simulink model "plant_fuzzy"  (R2020a)
settings: Solver=VariableStepAuto  StartTime=0.0  StopTime=200  RelTol=1e-3
values from neighbouring files (symbols this model uses):
  Ca = 0.005    [reproduce_examples.m]
  Cb = 0.005    [reproduce_examples.m]
  dt = 0.05    [reproduce_examples.m]
  fA = 2    [reproduce_examples.m]
  use_step = 1    [reproduce_examples.m]
  V = 3    [reproduce_examples.m]
libraries: simulink x2, fuzblock x1
settings Model: Creator=salvatore  LastModifiedBy=salvatore
settings DataIOCC: SaveFormat=Array  OutputSaveName=pH, valve

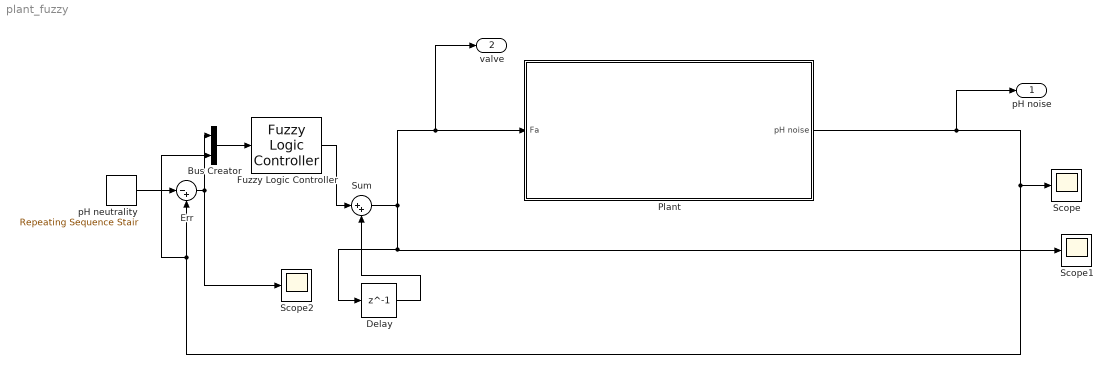
== system plant_fuzzy ==
  Bus Creator : BusCreator  Inputs=2
  Delay : Delay  DelayLength=1  InitialCondition=0
  Err : Sum  Inputs=|-+
  Fuzzy Logic Controller : fuzblock/Fuzzy Logic  Controller  FIS='fuzzy_ph.fis'  OutputSampleNumber=101  DataType=double  FuzzifiedInputs=off  RuleFiringStrengths=off  RuleOutputs=off  AggregatedOutputs=off  SimulateUsing=Interpreted execution  OutOfRangeInputValueMessage=warning  NoRuleFiredMessage=warning  EmptyOutputFuzzySetMessage=warning
  Plant : Subsystem
  Scope : Scope
  Scope1 : Scope
  Scope2 : Scope
  Sum : Sum  Inputs=|++
  pH neutrality : simulink/Sources/Repeating Sequence Stair  OutValues=reference  tsamp=time_ref  OutMin=[]  OutMax=[]  OutDataTypeStr=double  OutputDataTypeScalingMode=double  OutDataType=fixdt(0,8)  ConRadixGroup=Best Precision: Vector-wise  OutScaling=2^-12
  pH noise : Outport  SignalName=ph_noise
  valve : Outport  Port=2  SignalName=valve
  wires:
  pH neutrality/1 -> Err/1
  Sum/1 -> Delay/1, Scope1/1, valve/1, Plant/1(Fa)
  Fuzzy Logic Controller/1 -> Sum/1
  Delay/1 -> Sum/2
  Plant/1(pH noise) -> pH noise/1, Bus Creator/2, Err/2, Scope/1
  Err/1 -> Bus Creator/1, Scope2/1
  Bus Creator/1 -> Fuzzy Logic Controller/1

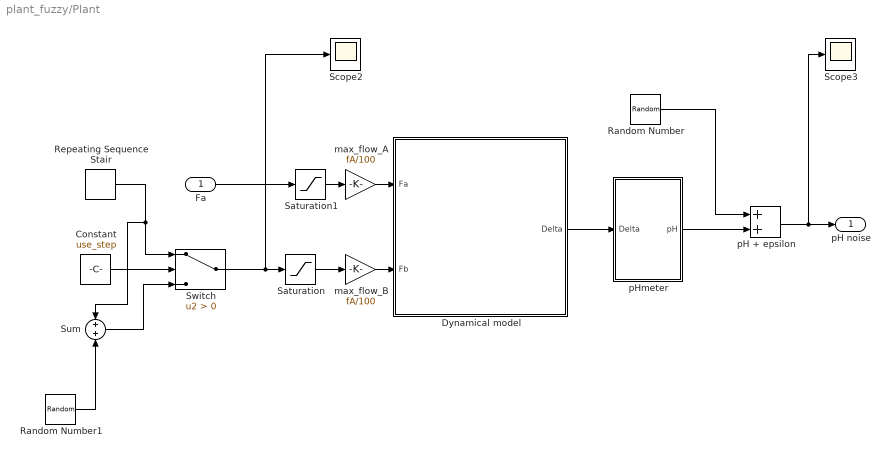
== system plant_fuzzy/Plant ==
  Fa : Inport
  Constant : Constant  Value=use_step
  Dynamical model : Subsystem
  Random Number : RandomNumber  Variance=0.01  SampleTime=dt
  Random Number1 : RandomNumber  Variance=4  SampleTime=1
  Repeating Sequence Stair : simulink/Sources/Repeating Sequence Stair  OutValues=out_valv  tsamp=time_valv  OutMin=[]  OutMax=[]  OutDataTypeStr=double  OutputDataTypeScalingMode=double  OutDataType=fixdt(0,8)  ConRadixGroup=Best Precision: Vector-wise  OutScaling=2^-12
  Saturation : Saturate  UpperLimit=100  LowerLimit=0
  Saturation1 : Saturate  UpperLimit=100  LowerLimit=0
  Scope2 : Scope
  Scope3 : Scope
  Sum : Sum  Inputs=+|+
  Switch : Switch  Criteria=u2 > Threshold
  max_flow_A : Gain  Gain=fA/100
  max_flow_B : Gain  Gain=fA/100
  pH + epsilon : Sum
  pHmeter : Subsystem
  pH noise : Outport
  wires:
  max_flow_A/1 -> Dynamical model/1(Fa)
  max_flow_B/1 -> Dynamical model/2(Fb)
  pH + epsilon/1 -> Scope3/1, pH noise/1
  pHmeter/1(pH) -> pH + epsilon/2
  Saturation1/1 -> max_flow_A/1
  Random Number/1 -> pH + epsilon/1
  Saturation/1 -> max_flow_B/1
  Dynamical model/1(Delta) -> pHmeter/1(Delta)
  Sum/1 -> Switch/3
  Constant/1 -> Switch/2
  Repeating Sequence Stair/1 -> Sum/1, Switch/1
  Fa/1 -> Saturation1/1
  Switch/1 -> Scope2/1, Saturation/1
  Random Number1/1 -> Sum/2

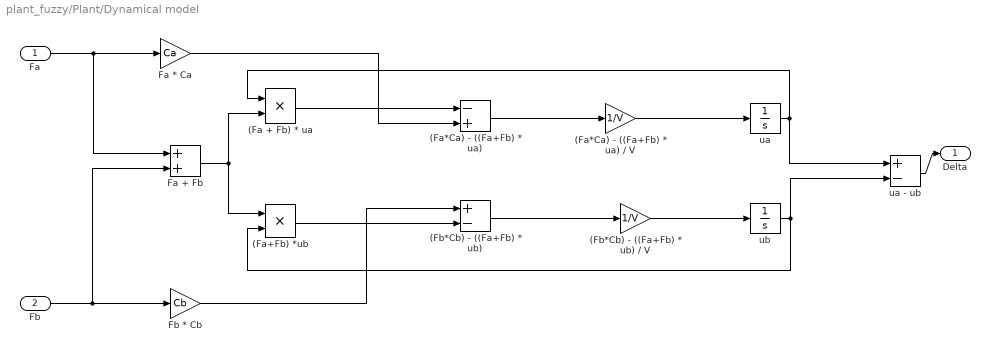
== system plant_fuzzy/Plant/Dynamical model ==
  Fa : Inport
  Fb : Inport  Port=2
  "(Fa + Fb) * ua " : Product  Inputs=**
  (Fa*Ca) - ((Fa+Fb) * ua) : Sum  Inputs=-+
  (Fa*Ca) - ((Fa+Fb) * ua) / V : Gain  Gain=1/V
  "(Fa+Fb) *ub  " : Product  Inputs=**
  (Fb*Cb) - ((Fa+Fb) * ub) : Sum  Inputs=+-
  (Fb*Cb) - ((Fa+Fb) * ub) / V : Gain  Gain=1/V
  "Fa * Ca " : Gain  Gain=Ca
  Fa + Fb : Sum
  Fb * Cb : Gain  Gain=Cb
  ua : Integrator  LimitOutput=on  UpperSaturationLimit=1  LowerSaturationLimit=0
  ua - ub : Sum  Inputs=+-
  ub : Integrator  LimitOutput=on  UpperSaturationLimit=1  LowerSaturationLimit=0
  Delta : Outport
  wires:
  (Fa*Ca) - ((Fa+Fb) * ua) / V/1 -> ua/1
  Fa/1 -> Fa + Fb/1, "Fa * Ca "/1
  "(Fa + Fb) * ua "/1 -> (Fa*Ca) - ((Fa+Fb) * ua)/1
  "Fa * Ca "/1 -> (Fa*Ca) - ((Fa+Fb) * ua)/2
  ub/1 -> ua - ub/2, "(Fa+Fb) *ub  "/2
  Fb/1 -> Fa + Fb/2, Fb * Cb/1
  Fb * Cb/1 -> (Fb*Cb) - ((Fa+Fb) * ub)/1
  "(Fa+Fb) *ub  "/1 -> (Fb*Cb) - ((Fa+Fb) * ub)/2
  Fa + Fb/1 -> "(Fa+Fb) *ub  "/1, "(Fa + Fb) * ua "/2
  (Fb*Cb) - ((Fa+Fb) * ub) / V/1 -> ub/1
  ua - ub/1 -> Delta/1
  ua/1 -> ua - ub/1, "(Fa + Fb) * ua "/1
  (Fa*Ca) - ((Fa+Fb) * ua)/1 -> (Fa*Ca) - ((Fa+Fb) * ua) / V/1
  (Fb*Cb) - ((Fa+Fb) * ub)/1 -> (Fb*Cb) - ((Fa+Fb) * ub) / V/1

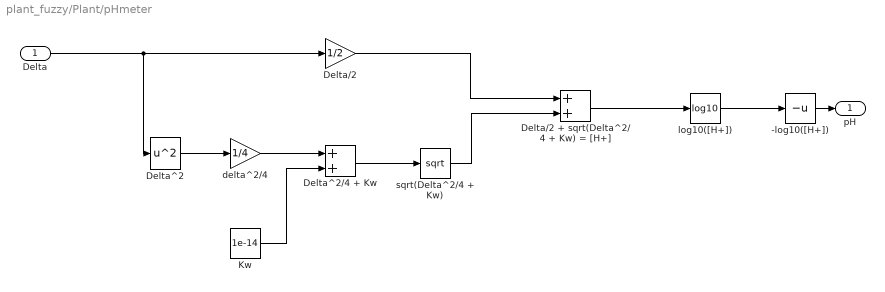
== system plant_fuzzy/Plant/pHmeter ==
  Delta : Inport
  -log10([H+]) : UnaryMinus
  Delta/2 : Gain  Gain=1/2
  Delta/2 + sqrt(Delta^2/4 + Kw) = [H+] : Sum
  Delta^2 : Math  Operator=square  SaturateOnIntegerOverflow=on
  Delta^2/4 + Kw : Sum
  Kw : Constant  Value=1e-14
  delta^2/4 : Gain  Gain=1/4
  "log10([H+]) " : Math  Operator=log10  SaturateOnIntegerOverflow=on
  sqrt(Delta^2/4 + Kw) : Sqrt  SaturateOnIntegerOverflow=on
  pH : Outport
  wires:
  "log10([H+]) "/1 -> -log10([H+])/1
  Delta^2/4 + Kw/1 -> sqrt(Delta^2/4 + Kw)/1
  -log10([H+])/1 -> pH/1
  Kw/1 -> Delta^2/4 + Kw/2
  sqrt(Delta^2/4 + Kw)/1 -> Delta/2 + sqrt(Delta^2/4 + Kw) = [H+]/2
  Delta/2 + sqrt(Delta^2/4 + Kw) = [H+]/1 -> "log10([H+]) "/1
  Delta/1 -> Delta/2/1, Delta^2/1
  Delta^2/1 -> delta^2/4/1
  delta^2/4/1 -> Delta^2/4 + Kw/1
  Delta/2/1 -> Delta/2 + sqrt(Delta^2/4 + Kw) = [H+]/1
